simulink model "thrityonelevel_inverter"  (Simulink 10.3)
settings: Solver=ode45  StartTime=0.0  StopTime=2  RelTol=1e-3  EnableMultiTasking=on
libraries: simulink x32, spsIGBTDiodeLib x12, spsVoltageMeasurementLib x11, spsDCVoltageSourceLib x4, spsSeriesRLCBranchLib x1, spspowerguiLib x1
settings Model: Creator=abdul haleem  LastModifiedBy=rtras  MultithreadedSim=on
settings DataIOCC: LimitDataPoints=on
settings DebuggingCC: SolverPrmCheckMsg=warning

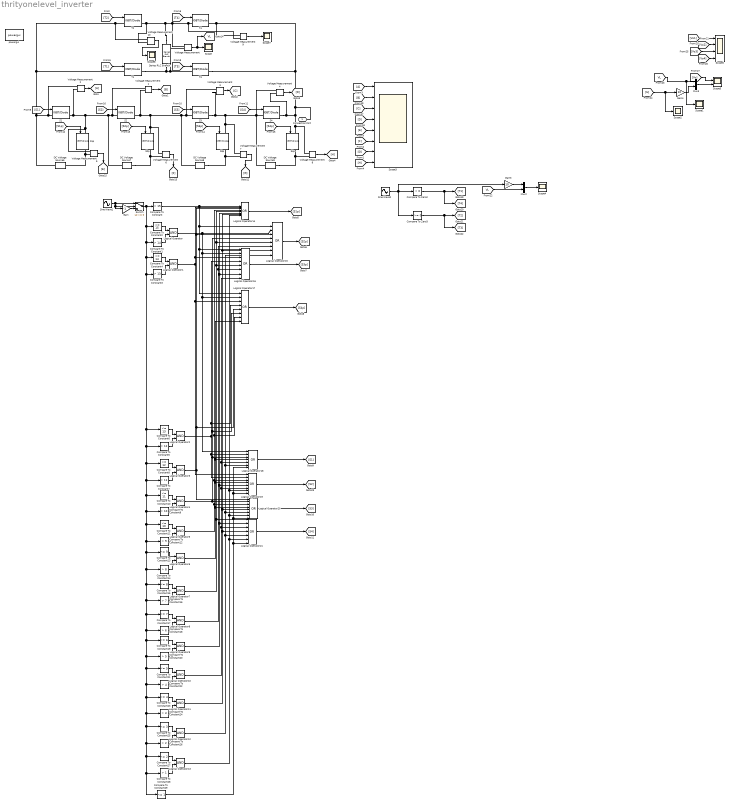
== system thrityonelevel_inverter ==
  Compare To Constant : simulink/Logic and Bit Operations/Compare To Constant  relop=>  const=15  OutDataTypeStr=uint8  ZeroCross=off
  Compare To Constant1 : simulink/Logic and Bit Operations/Compare To Constant  relop=>  const=14  OutDataTypeStr=uint8  ZeroCross=off
  Compare To Constant10 : simulink/Logic and Bit Operations/Compare To Constant  relop=<=  const=11  OutDataTypeStr=uint8  ZeroCross=off
  Compare To Constant11 : simulink/Logic and Bit Operations/Compare To Constant  relop=<=  const=10  OutDataTypeStr=uint8  ZeroCross=off
  Compare To Constant12 : simulink/Logic and Bit Operations/Compare To Constant  relop=>  const=9  OutDataTypeStr=uint8  ZeroCross=off
  Compare To Constant13 : simulink/Logic and Bit Operations/Compare To Constant  relop=<=  const=9  OutDataTypeStr=uint8  ZeroCross=off
  Compare To Constant14 : simulink/Logic and Bit Operations/Compare To Constant  relop=>  const=8  OutDataTypeStr=uint8  ZeroCross=off
  Compare To Constant15 : simulink/Logic and Bit Operations/Compare To Constant  relop=<=  const=8  OutDataTypeStr=uint8  ZeroCross=off
  Compare To Constant16 : simulink/Logic and Bit Operations/Compare To Constant  relop=>  const=7  OutDataTypeStr=uint8  ZeroCross=off
  Compare To Constant17 : simulink/Logic and Bit Operations/Compare To Constant  relop=<=  const=7  OutDataTypeStr=uint8  ZeroCross=off
  Compare To Constant18 : simulink/Logic and Bit Operations/Compare To Constant  relop=>  const=6  OutDataTypeStr=uint8  ZeroCross=off
  Compare To Constant19 : simulink/Logic and Bit Operations/Compare To Constant  relop=<=  const=6  OutDataTypeStr=uint8  ZeroCross=off
  Compare To Constant2 : simulink/Logic and Bit Operations/Compare To Constant  relop=<=  const=15  OutDataTypeStr=uint8  ZeroCross=off
  Compare To Constant20 : simulink/Logic and Bit Operations/Compare To Constant  relop=>  const=5  OutDataTypeStr=uint8  ZeroCross=off
  Compare To Constant21 : simulink/Logic and Bit Operations/Compare To Constant  relop=<=  const=5  OutDataTypeStr=uint8  ZeroCross=off
  Compare To Constant22 : simulink/Logic and Bit Operations/Compare To Constant  relop=>  const=4  OutDataTypeStr=uint8  ZeroCross=off
  Compare To Constant23 : simulink/Logic and Bit Operations/Compare To Constant  relop=<=  const=4  OutDataTypeStr=uint8  ZeroCross=off
  Compare To Constant24 : simulink/Logic and Bit Operations/Compare To Constant  relop=>  const=3  OutDataTypeStr=uint8  ZeroCross=off
  Compare To Constant25 : simulink/Logic and Bit Operations/Compare To Constant  relop=<=  const=3  OutDataTypeStr=uint8  ZeroCross=off
  Compare To Constant26 : simulink/Logic and Bit Operations/Compare To Constant  relop=>  const=2  OutDataTypeStr=uint8  ZeroCross=off
  Compare To Constant27 : simulink/Logic and Bit Operations/Compare To Constant  relop=<=  const=2  OutDataTypeStr=uint8  ZeroCross=off
  Compare To Constant28 : simulink/Logic and Bit Operations/Compare To Constant  relop=>  const=1  OutDataTypeStr=uint8  ZeroCross=off
  Compare To Constant29 : simulink/Logic and Bit Operations/Compare To Constant  relop=<=  const=1  OutDataTypeStr=uint8  ZeroCross=off
  Compare To Constant3 : simulink/Logic and Bit Operations/Compare To Constant  relop=>  const=13  OutDataTypeStr=uint8  ZeroCross=off
  Compare To Constant4 : simulink/Logic and Bit Operations/Compare To Constant  relop=<=  const=14  OutDataTypeStr=uint8  ZeroCross=off
  Compare To Constant5 : simulink/Logic and Bit Operations/Compare To Constant  relop=>  const=12  OutDataTypeStr=uint8  ZeroCross=off
  Compare To Constant6 : simulink/Logic and Bit Operations/Compare To Constant  relop=<=  const=13  OutDataTypeStr=uint8  ZeroCross=off
  Compare To Constant7 : simulink/Logic and Bit Operations/Compare To Constant  relop=>  const=11  OutDataTypeStr=uint8  ZeroCross=off
  Compare To Constant8 : simulink/Logic and Bit Operations/Compare To Constant  relop=<=  const=12  OutDataTypeStr=uint8  ZeroCross=off
  Compare To Constant9 : simulink/Logic and Bit Operations/Compare To Constant  relop=>  const=10  OutDataTypeStr=uint8  ZeroCross=off
  Compare To Zero2 : simulink/Logic and Bit Operations/Compare To Zero  relop=<  OutDataTypeStr=uint8  ZeroCross=off
  Compare To Zero3 : simulink/Logic and Bit Operations/Compare To Zero  relop=>=  OutDataTypeStr=uint8  ZeroCross=off
  DC Voltage Source6 : spsDCVoltageSourceLib/DC Voltage Source  Amplitude=15  Measurements=None
  DC Voltage Source7 : spsDCVoltageSourceLib/DC Voltage Source  Amplitude=30  Measurements=None
  DC Voltage Source8 : spsDCVoltageSourceLib/DC Voltage Source  Amplitude=60  Measurements=None
  DC Voltage Source9 : spsDCVoltageSourceLib/DC Voltage Source  Amplitude=120  Measurements=None
  Gain : Gain  Gain=-1
  Gain3 : Gain  Gain=10
  Gain4 : Gain  Gain=10
  Logical Operator{,1..13} (14 alike) : Logic  AllPortsSameDT=off  OutDataTypeStr=boolean
  Logical Operator{14..17,19..20} (6 alike) : Logic  Operator=OR  Inputs=8  AllPortsSameDT=off  OutDataTypeStr=boolean
  Logical Operator18 : Logic  Operator=OR  Inputs=7  AllPortsSameDT=off  OutDataTypeStr=boolean
  Logical Operator21 : Logic  Operator=OR  Inputs=7  AllPortsSameDT=off  OutDataTypeStr=boolean
  Mux2 : Mux  Inputs=2
  Mux3 : Mux  Inputs=2
  S{1..4} (4 alike) : spsIGBTDiodeLib/IGBT//Diode  Ron=1e-3  Rs=1e5  Cs=inf  Measurements=on
  S1p : spsIGBTDiodeLib/IGBT//Diode  Ron=1e-3  Rs=1e5  Cs=inf  Measurements=on
  S2p : spsIGBTDiodeLib/IGBT//Diode  Ron=1e-3  Rs=1e5  Cs=inf  Measurements=on
  S3p : spsIGBTDiodeLib/IGBT//Diode  Ron=1e-3  Rs=1e5  Cs=inf  Measurements=on
  S4p : spsIGBTDiodeLib/IGBT//Diode  Ron=1e-3  Rs=1e5  Cs=inf  Measurements=on
  Scope{,1..2,4,7..8} (6 alike) : Scope
  Scope3 : Scope  NumInputPorts=8
  Scope5 : Scope  NumInputPorts=2
  Scope6 : Scope  NumInputPorts=4
  Series RLC Branch : spsSeriesRLCBranchLib/Series RLC Branch  LConnTagsString=__new0  RConnTagsString=__new0  BranchType=RL  Resistance=45  Inductance=55e-3  SetiL0=off  InitialCurrent=0  Capacitance=1e-6  Setx0=off  InitialVoltage=0  Measurements=None
  Sine Wave1 : Sin  Amplitude=16  Frequency=2*pi*50  SampleTime=0
  Sine Wave2 : Sin  Amplitude=15  Frequency=2*pi*50  SampleTime=0
  Switch : Switch
  T{1..4} (4 alike) : spsIGBTDiodeLib/IGBT//Diode  Ron=1e-3  Rs=1e5  Cs=inf  Measurements=on
  Voltage Measurement{,1..10} (11 alike) : spsVoltageMeasurementLib/Voltage Measurement  PhasorSimulation=off  OutputType=Complex  PSBequivalent=0
  powergui : spspowerguiLib/powergui  Priority=1  SimulationMode=Discrete  SampleTime=50e-6  frequency=60  Iterations=50  frequencyindice=0  Pbase=100e6  ErrMax=1e-4  UnitsV=kV  UnitsW=MW  buscounter=0  FunctionMessages=off  echomessages=off  EnableUseOfTLC=off  CurrentSourceSwitches=off  DisableSnubberDevices=off  DisableRonSwitches=off  DisableVfSwitches=off  DisplayEquations=off  AutomaticDiscreteSolvers=off  SolverType=Tustin/Backward Euler (TBE)  Interpol=off  ExternalGateDelay=off  methode=off  Ts=0  x0status=blocks  SPID=off  SwTol=0  HookPort=off  NonlinearTolerance=1e-4  nMaxIteration=100  ContinueOnMaxIteration=off  RestoreLinks=warning  ResistiveCurrentMeasurement=off  Frange=[0:2:500]  Ylog=off  Xlog=on  ShowGrid=off  save=off  variable=ZData  structure=ScopeData4  ZoomFFT=off  StartTime=0.0  cycles=25  DisplayStyle=3  fundamental=50  FreqAxis=on  MaxFrequency=1000  frequencyindicesteady=1  RmsSteady=1  display=off
  Connection Port : PMIOPort  Side=Left
  tag scope: VL=global
  wires:
  [T2] -> T2/1
  [T1] -> T1/1
  [T4] -> T4/1
  [T3] -> T3/1
  Voltage Measurement/1 -> Scope/1, [VL]
  [S1] -> S1/1
  [S1p] -> S1p/1
  [S2p] -> S2p/1
  [S3p] -> S3p/1
  [S4p] -> S4p/1
  [S2] -> S2/1
  [S3] -> S3/1
  [S4] -> S4/1
  Sine Wave2/1 -> Compare To Zero2/1, Compare To Zero3/1, Gain3/1
  Compare To Zero2/1 -> [T1], [T4]
  Compare To Zero3/1 -> [T3], [T2]
  [VL] -> Mux2/2
  Mux2/1 -> Scope4/1
  Gain/1 -> Switch/3
  Switch/1 -> Compare To Constant/1, Compare To Constant2/1, Compare To Constant1/1, Compare To Constant4/1, Compare To Constant3/1, Compare To Constant6/1, Compare To Constant5/1, Compare To Constant8/1, Compare To Constant7/1, Compare To Constant10/1, Compare To Constant9/1, Compare To Constant11/1, Compare To Constant12/1, Compare To Constant13/1, Compare To Constant14/1, Compare To Constant15/1, Compare To Constant16/1, Compare To Constant17/1, Compare To Constant18/1, Compare To Constant19/1, Compare To Constant20/1, Compare To Constant21/1, Compare To Constant22/1, Compare To Constant23/1, Compare To Constant24/1, Compare To Constant25/1, Compare To Constant26/1, Compare To Constant27/1, Compare To Constant28/1, Compare To Constant29/1
  Compare To Constant2/1 -> Logical Operator/1
  Compare To Constant1/1 -> Logical Operator/2
  Compare To Constant4/1 -> Logical Operator1/1
  Compare To Constant3/1 -> Logical Operator1/2
  Compare To Constant6/1 -> Logical Operator2/1
  Compare To Constant5/1 -> Logical Operator2/2
  Logical Operator2/1 -> Logical Operator18/2, Logical Operator19/2, Logical Operator16/4, Logical Operator17/4
  Compare To Constant8/1 -> Logical Operator3/1
  Compare To Constant7/1 -> Logical Operator3/2
  Compare To Constant10/1 -> Logical Operator4/1
  Compare To Constant9/1 -> Logical Operator4/2
  Sine Wave1/1 -> Switch/1, Switch/2, Gain/1
  Compare To Constant11/1 -> Logical Operator5/1
  Compare To Constant12/1 -> Logical Operator5/2
  Compare To Constant13/1 -> Logical Operator6/1
  Compare To Constant14/1 -> Logical Operator6/2
  Compare To Constant15/1 -> Logical Operator7/1
  Compare To Constant16/1 -> Logical Operator7/2
  Compare To Constant17/1 -> Logical Operator8/1
  Compare To Constant18/1 -> Logical Operator8/2
  Compare To Constant19/1 -> Logical Operator9/1
  Compare To Constant20/1 -> Logical Operator9/2
  Compare To Constant21/1 -> Logical Operator10/1
  Compare To Constant22/1 -> Logical Operator10/2
  Compare To Constant23/1 -> Logical Operator11/1
  Compare To Constant24/1 -> Logical Operator11/2
  Compare To Constant25/1 -> Logical Operator12/1
  Compare To Constant26/1 -> Logical Operator12/2
  Compare To Constant27/1 -> Logical Operator13/1
  Compare To Constant28/1 -> Logical Operator13/2
  Logical Operator14/1 -> [S1p]
  Logical Operator15/1 -> [S2p]
  Logical Operator16/1 -> [S3p]
  Logical Operator17/1 -> [S4p]
  Logical Operator18/1 -> [S1]
  Logical Operator19/1 -> [S2]
  Logical Operator20/1 -> [S3]
  Logical Operator21/1 -> [S4]
  Compare To Constant/1 -> Logical Operator14/1, Logical Operator15/1, Logical Operator16/1, Logical Operator17/1
  Logical Operator/1 -> Logical Operator15/2, Logical Operator16/2, Logical Operator17/2, Logical Operator18/1
  Logical Operator1/1 -> Logical Operator14/2, Logical Operator16/3, Logical Operator17/3, Logical Operator19/1
  Logical Operator3/1 -> Logical Operator14/3, Logical Operator15/3, Logical Operator17/5, Logical Operator20/1
  Logical Operator4/1 -> Logical Operator15/4, Logical Operator17/6, Logical Operator18/3, Logical Operator20/2
  Logical Operator5/1 -> Logical Operator14/4, Logical Operator17/7, Logical Operator19/3, Logical Operator20/3
  Logical Operator6/1 -> Logical Operator17/8, Logical Operator18/4, Logical Operator19/4, Logical Operator20/4
  Logical Operator7/1 -> Logical Operator21/1, Logical Operator14/5, Logical Operator15/5, Logical Operator16/5
  Logical Operator8/1 -> Logical Operator15/6, Logical Operator16/6
  Logical Operator9/1 -> Logical Operator14/6, Logical Operator16/7, Logical Operator19/5, Logical Operator21/2
  Logical Operator10/1 -> Logical Operator21/3, Logical Operator19/6, Logical Operator18/5, Logical Operator16/8
  Logical Operator11/1 -> Logical Operator21/4, Logical Operator20/5, Logical Operator14/7, Logical Operator15/7
  Logical Operator12/1 -> Logical Operator21/5, Logical Operator20/6, Logical Operator18/6, Logical Operator15/8
  Logical Operator13/1 -> Logical Operator21/6, Logical Operator20/7, Logical Operator19/7, Logical Operator14/8
  Compare To Constant29/1 -> Logical Operator21/7, Logical Operator20/8, Logical Operator19/8, Logical Operator18/7
  Gain3/1 -> Mux2/1
  [Vo1] -> Scope6/1
  [Vo2] -> Scope6/2
  [Vo3] -> Scope6/3
  [Vo4] -> Scope6/4
  Mux3/1 -> Scope5/2
  [VL] -> Mux3/1, Scope1/1
  [IL] -> Gain4/1, Scope2/1
  Gain4/1 -> Mux3/2
  [Vo] -> Scope5/1
  [A] -> Scope3/1
  [B] -> Scope3/2
  [C] -> Scope3/3
  [D] -> Scope3/4
  [E] -> Scope3/5
  [F] -> Scope3/6
  [G] -> Scope3/7
  [H] -> Scope3/8
  Voltage Measurement2/1 -> [A]
  Voltage Measurement1/1 -> [B]
  Voltage Measurement3/1 -> [C]
  Voltage Measurement4/1 -> [D]
  Voltage Measurement8/1 -> [H]
  Voltage Measurement7/1 -> [G]
  Voltage Measurement6/1 -> [F]
  Voltage Measurement5/1 -> [E]
  Voltage Measurement9/1 -> Scope7/1
  Voltage Measurement10/1 -> Scope8/1
  connections:
  Series RLC Branch/LConn1 -- Voltage Measurement10/LConn2 -- T2/RConn1 -- Voltage Measurement/LConn1 -- Voltage Measurement9/LConn2 -- T4/LConn1
  T1/RConn1 -- Series RLC Branch/RConn1 -- T3/LConn1 -- Voltage Measurement/LConn2
  T1/LConn1 -- Voltage Measurement10/LConn1 -- T2/LConn1 -- DC Voltage Source6/RConn1 -- Voltage Measurement2/LConn1 -- S1/LConn1
  Connection Port/RConn1 -- Voltage Measurement4/LConn2 -- S4/RConn1 -- Voltage Measurement8/LConn1 -- S4p/LConn1 -- T3/RConn1 -- Voltage Measurement9/LConn1 -- T4/RConn1
  DC Voltage Source7/RConn1 -- Voltage Measurement2/LConn2 -- S1/RConn1 -- Voltage Measurement5/LConn1 -- S1p/LConn1 -- Voltage Measurement1/LConn1 -- S2/LConn1
  Voltage Measurement6/LConn1 -- S2p/LConn1 -- DC Voltage Source8/RConn1 -- Voltage Measurement3/LConn1 -- S3/LConn1 -- Voltage Measurement1/LConn2 -- S2/RConn1
  Voltage Measurement3/LConn2 -- S3/RConn1 -- Voltage Measurement7/LConn1 -- S3p/LConn1 -- Voltage Measurement4/LConn1 -- DC Voltage Source9/RConn1 -- S4/LConn1
  DC Voltage Source7/LConn1 -- Voltage Measurement6/LConn2 -- S2p/RConn1
  S1p/RConn1 -- DC Voltage Source6/LConn1 -- Voltage Measurement5/LConn2
  DC Voltage Source9/LConn1 -- Voltage Measurement8/LConn2 -- S4p/RConn1
  DC Voltage Source8/LConn1 -- Voltage Measurement7/LConn2 -- S3p/RConn1
